simulink model "underwater_gen_1"  (R2021a)
settings: Solver=VariableStepAuto  StartTime=0.0  StopTime=24  RelTol=1e-3
libraries: spsACVoltageSourceLib x3, spsGroundLib x1, spsWindTurbineInductionGeneratorPhasorTypeLib x1, spspowerguiLib x1
settings Model: Creator=siddh  LastModifiedBy=siddh

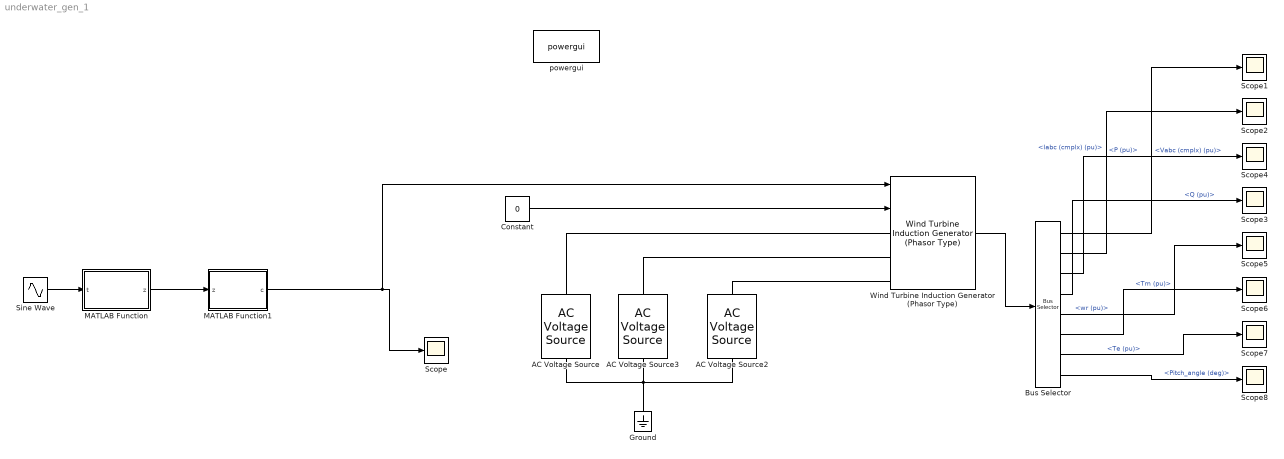
== system underwater_gen_1 ==
  AC Voltage Source : spsACVoltageSourceLib/AC Voltage Source  Amplitude=325.27  Phase=0  Frequency=50  SampleTime=0.001  Measurements=None  BusType=swing  Pref=10e3  Qref=0  Qmin=-inf  Qmax=+inf
  AC Voltage Source2 : spsACVoltageSourceLib/AC Voltage Source  Amplitude=325.27  Phase=240  Frequency=50  SampleTime=0.001  Measurements=None  BusType=swing  Pref=10e3  Qref=0  Qmin=-inf  Qmax=+inf
  AC Voltage Source3 : spsACVoltageSourceLib/AC Voltage Source  Amplitude=325.27  Phase=120  Frequency=50  SampleTime=0.001  Measurements=None  BusType=swing  Pref=10e3  Qref=0  Qmin=-inf  Qmax=+inf
  Bus Selector : BusSelector  OutputSignals=Vabc (cmplx) (pu),Iabc (cmplx) (pu),P (pu),Q (pu),wr (pu),Tm (pu),Te (pu),Pitch_angle (deg)
  Constant : Constant  Value=0
  Ground : spsGroundLib/Ground  LConnTagsString=a
  MATLAB Function : MATLAB Function  TreatAsAtomicUnit=on
  MATLAB Function1 : MATLAB Function  TreatAsAtomicUnit=on
  Scope{,1..8} (9 alike) : Scope
  Sine Wave : Sin  Amplitude=4  Frequency=2*pi*1/14  SampleTime=0.001
  Wind Turbine Induction Generator (Phasor Type) : spsWindTurbineInductionGeneratorPhasorTypeLib/Wind Turbine Induction Generator (Phasor Type)  ExternalTm=off  nom=[1.5e6/0.9, 575, 50]  sta=[ 0.004843, 0.1248]  rot=[ 0.004377, 0.1791]  Lm=6.77  mec=[5.04, 0.01, 3]  init="[ -0.01,0,   0,0,0,   0,0,0 ]"  pitch_angle=0  Pmec=1.5e6  wind_base=4  speed_nom=1  P_wind_base=3e6  K_pitch_gain=[0 0]  pitch_max=35  pitch_rate=0
      settings: SourceProductBaseCode=PS
  powergui : spspowerguiLib/powergui  Priority=1  SimulationMode=Continuous  SampleTime=50e-6  frequency=60  Iterations=50  frequencyindice=50  Pbase=100e6  ErrMax=1e-4  UnitsV=kV  UnitsW=MW  buscounter=0  FunctionMessages=off  echomessages=off  EnableUseOfTLC=off  CurrentSourceSwitches=off  DisableSnubberDevices=off  DisableRonSwitches=off  DisableVfSwitches=off  DisplayEquations=off  AutomaticDiscreteSolvers=off  SolverType=Tustin/Backward Euler (TBE)  Interpol=off  ExternalGateDelay=off  methode=off  Ts=100  x0status=blocks  SPID=on  SwTol=0  HookPort=off  NonlinearTolerance=1e-4  nMaxIteration=100  ContinueOnMaxIteration=off  RestoreLinks=warning  ResistiveCurrentMeasurement=off  Frange=[0:2:500]  Ylog=off  Xlog=on  ShowGrid=off  save=off  variable=ZData  structure=0  ZoomFFT=off  StartTime=0.0  cycles=1  DisplayStyle=1  fundamental=60  FreqAxis=off  MaxFrequency=1000  frequencyindicesteady=1  RmsSteady=1  display=off
  wires:
  Sine Wave/1 -> MATLAB Function/1(t)
  MATLAB Function1/1(c) -> Wind Turbine Induction Generator (Phasor Type)/1, Scope/1
  MATLAB Function/1(z) -> MATLAB Function1/1(z)
  Wind Turbine Induction Generator (Phasor Type)/1 -> Bus Selector/1
  Constant/1 -> Wind Turbine Induction Generator (Phasor Type)/2
  Bus Selector/1 -> Scope1/1  "<Vabc (cmplx) (pu)>"
  Bus Selector/2 -> Scope2/1  "<Iabc (cmplx) (pu)>"
  Bus Selector/3 -> Scope4/1  "<P (pu)>"
  Bus Selector/4 -> Scope3/1  "<Q (pu)>"
  Bus Selector/5 -> Scope5/1  "<wr (pu)>"
  Bus Selector/6 -> Scope6/1  "<Tm (pu)>"
  Bus Selector/7 -> Scope7/1  "<Te (pu)>"
  Bus Selector/8 -> Scope8/1  "<Pitch_angle (deg)>"
  connections:
  AC Voltage Source/RConn1 -- Wind Turbine Induction Generator (Phasor Type)/LConn1
  AC Voltage Source2/RConn1 -- Wind Turbine Induction Generator (Phasor Type)/LConn3
  AC Voltage Source3/RConn1 -- Wind Turbine Induction Generator (Phasor Type)/LConn2
  Ground/LConn1 -- AC Voltage Source3/LConn1 -- AC Voltage Source2/LConn1 -- AC Voltage Source/LConn1

== matlab function underwater_gen_1/MATLAB Function ==
  data: t input; z output
function z = speed_of_waves(t)

z = abs(t);

end

== matlab function underwater_gen_1/MATLAB Function1 ==
  data: z input; c output
function c = clipper(z)

if(z>=4)
   c = 4;

else
    c = z;
end

end
